simulink model "autopilot_vtolsim"  (R2019a)
settings: Solver=ode15s  StartTime=0.0  StopTime=10000  RelTol=1e-3  EnableMultiTasking=on
InitFcn:
  | clear all
  | path(pathdef)
  | addpath('.')
  | simulation_parameters
  | wind_parameters
undefined symbols (not defined in the file or in its folder): AP, autopilot, drawAircraft, Earth, forces_moments, plotvtolstatevariables, SIM, true_states, vtol, WGS84, WIND
libraries: simulink x3, aerolibfltsims x2, aerolibtransform2 x1
settings Model: Creator=beard  LastModifiedBy=nikhil
settings DataIOCC: LimitDataPoints=on  SaveFormat=Array  SignalLoggingSaveFormat=ModelDataLogs  ReturnWorkspaceOutputs=off
settings OptimizationCC: ExpressionDepthLimit=2147483647  InitFltsAndDblsToZero=on  LifeSpan=inf
settings DebuggingCC: UnderspecifiedInitializationDetection=Classic  MergeDetectMultiDrivingBlocksExec=none  SolverPrmCheckMsg=warning  FcnCallInpInsideContextMsg=warning  AllowSymbolicDim=off  StateNameClashWarn=warning  PregeneratedLibrarySubsystemCodeDiagnostic=none  SFUnexpectedBacktrackingDiag=warning  SFNoUnconditionalDefaultTransitionDiag=warning  SFExecutionAtInitializationDiag=none  ArithmeticOperatorsInVariantConditions=warning
settings HardwareCC: ProdBitPerPointer=32  ProdBitPerSizeT=32  ProdBitPerPtrDiffT=32  ProdLargestAtomicFloat=None  ProdIntDivRoundTo=Undefined  ProdEndianess=Unspecified  ProdWordSize=32  ProdHWDeviceType=32-bit Generic
settings ModelReferenceCC: PropagateSignalLabelsOutOfModel=off
settings SFSimCC: SimUseLocalCustomCode=off
settings RTWCC: RTWUseLocalCustomCode=off
settings CodeAppCC: StateflowObjectComments=on
settings GRTTargetCC: TargetLangStandard=C89/C90 (ANSI)  GeneratePreprocessorConditionals=Disable all  CombineOutputUpdateFcns=off  GRTInterface=on
settings ConfigComp: CovMetricSettings=dw  CovHtmlReporting=on  CovSaveCumulativeToWorkspaceVar=on  CovSaveSingleToWorkspaceVar=on  CovExternalEMLEnable=off  CovSFcnEnable=off

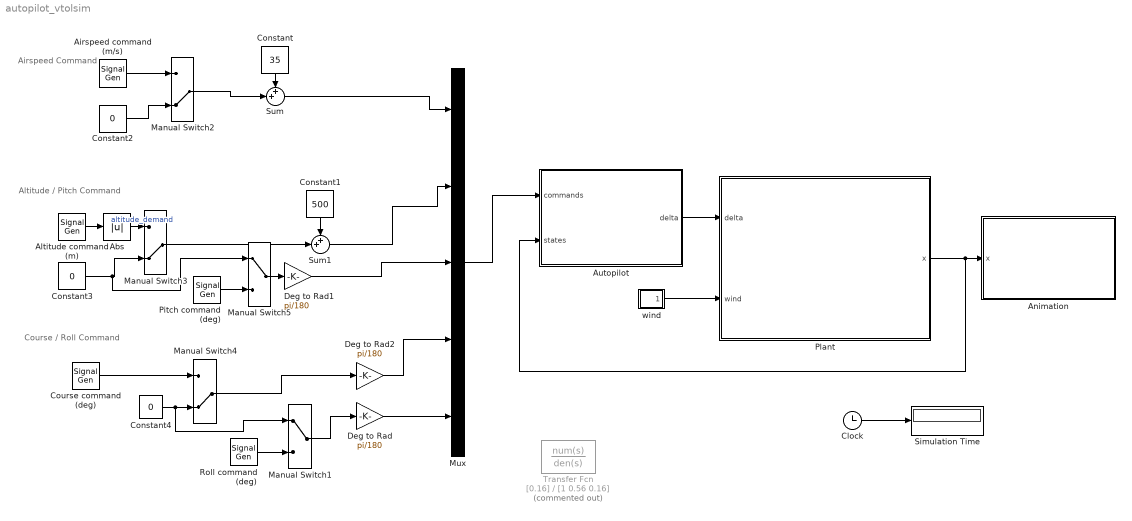
== system autopilot_vtolsim ==
  note: Airspeed Command
  note: Altitude / Pitch Command
  note: Course / Roll Command
  Abs : Abs
  Airspeed command (m/s) : SignalGenerator  WaveForm=square  Amplitude=5  Frequency=0.012
  Altitude command (m) : SignalGenerator  Amplitude=15  Frequency=.02
  Animation : Subsystem
      mask Display: image(imread('animation.jpg'))
  Autopilot : Subsystem
      mask Display: image(imread('stm32.jpg'))
  Clock : Clock
  Constant : Constant  Value=35
  Constant1 : Constant  Value=500
  Constant2 : Constant  Value=0
  Constant3 : Constant  Value=0
  Constant4 : Constant  Value=0
  Course command (deg) : SignalGenerator  Amplitude=45  Frequency=.012
  Deg to Rad : Gain  Gain=pi/180
  Deg to Rad1 : Gain  Gain=pi/180
  Deg to Rad2 : Gain  Gain=pi/180
  Manual Switch1 : ManualSwitch
  Manual Switch2 : ManualSwitch  CurrentSetting=0
  Manual Switch3 : ManualSwitch  CurrentSetting=0
  Manual Switch4 : ManualSwitch  CurrentSetting=0
  Manual Switch5 : ManualSwitch
  Mux : Mux  Inputs=5
  Pitch command (deg) : SignalGenerator  Amplitude=20  Frequency=0.1
  Plant : Subsystem
      mask Display: image(imread('vtol.jpeg'))
  Roll command (deg) : SignalGenerator  WaveForm=square  Amplitude=45  Frequency=.1
  Simulation Time : Display
  Sum : Sum  Inputs=++|
  Sum1 : Sum  Inputs=++|
  Transfer Fcn : TransferFcn  Commented=on  Numerator=[0.16]  Denominator=[1 0.56 0.16]
  wind : Subsystem
  wires:
  Clock/1 -> Simulation Time/1
  wind/1(Wind) -> Plant/2(wind)
  Plant/1(x) -> Autopilot/2(states), Animation/1(x)
  Autopilot/1(delta) -> Plant/1(delta)
  Deg to Rad/1 -> Mux/5
  Sum/1 -> Mux/1
  Constant/1 -> Sum/1
  Sum1/1 -> Mux/2
  Constant1/1 -> Sum1/1
  Deg to Rad1/1 -> Mux/3
  Airspeed command (m/s)/1 -> Manual Switch2/1
  Constant2/1 -> Manual Switch2/2
  Manual Switch3/1 -> Sum1/2
  Constant3/1 -> Manual Switch5/1, Manual Switch3/2
  Constant4/1 -> Manual Switch1/1, Manual Switch4/2
  Manual Switch4/1 -> Deg to Rad2/1
  Course command (deg)/1 -> Manual Switch4/1
  Manual Switch2/1 -> Sum/2
  Deg to Rad2/1 -> Mux/4
  Mux/1 -> Autopilot/1(commands)
  Roll command (deg)/1 -> Manual Switch1/2
  Manual Switch1/1 -> Deg to Rad/1
  Manual Switch5/1 -> Deg to Rad1/1
  Pitch command (deg)/1 -> Manual Switch5/2
  Altitude command (m)/1 -> Abs/1
  Abs/1 -> Manual Switch3/1  "altitude_demand"

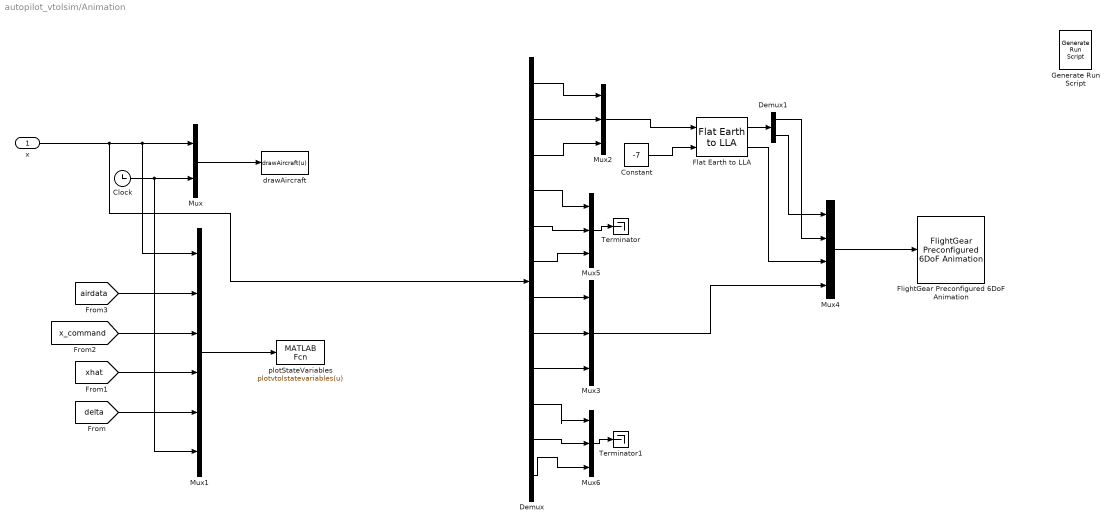
== system autopilot_vtolsim/Animation ==
  x : Inport
  Clock : Clock
  Constant : Constant  Value=-7
  Demux : Demux  Outputs=12
  Demux1 : Demux  Outputs=2
  Flat Earth to LLA : aerolibtransform2/Flat Earth to LLA  units=Metric (MKS)  ptype=Earth (WGS84)  F=1/298.257223563  R=6378137  LL0=[37.6188056,-122.3754167 ]  psi=0
  FlightGear Preconfigured 6DoF Animation : aerolibfltsims/FlightGear Preconfigured 6DoF Animation  xFlightGearVersion=v2018.2  DestinationIpAddress=127.0.0.1  DestinationPort=5502  SampleTime=1/30  packetVersion=24
      settings: SourceProductName=Aerospace Blockset
  Generate Run Script : aerolibfltsims/Generate Run Script  Architecture=Win64  dataFlow=Send  GeometryModelName=c172p  AirportId=KSFO  RunwayId=10L  InitialAltitude=0  InitialHeading=113  OffsetDistance=4.72  OffsetAzimuth=0  InstallScenery=on  DisableShaders=off  OriginAddress=127.0.0.1  DestinationPort=5502  OriginPort=5505  LocalAddress=127.0.0.1  OutputFileName=runfg.bat  FlightGearBaseDirectory=C:\Program Files\FlightGear 2019.1.1
  Mux : Mux  Inputs=2
  Mux1 : Mux  Inputs=6
  Mux{2..3,5..6} (4 alike) : Mux  Inputs=3
  Mux4 : Mux
  Terminator : Terminator
  Terminator1 : Terminator
  drawAircraft : MATLABFcn  MATLABFcn=drawAircraft(u)  OutputDimensions=0  SampleTime=SIM.ts_plotting
  plotStateVariables : MATLABFcn  MATLABFcn=plotvtolstatevariables(u)  OutputDimensions=0  SampleTime=SIM.ts_plotting
  wires:
  Mux/1 -> drawAircraft/1
  x/1 -> Demux/1, Mux/1, Mux1/1
  Clock/1 -> Mux/2, Mux1/6
  Mux1/1 -> plotStateVariables/1
  [xhat] -> Mux1/4
  [x_command] -> Mux1/3
  [delta] -> Mux1/5
  [airdata] -> Mux1/2
  Demux/1 -> Mux2/1
  Demux/2 -> Mux2/2
  Demux/3 -> Mux2/3
  Mux2/1 -> Flat Earth to LLA/1
  Constant/1 -> Flat Earth to LLA/2
  Demux/4 -> Mux5/1
  Demux/5 -> Mux5/2
  Demux/6 -> Mux5/3
  Demux/7 -> Mux3/1
  Demux/8 -> Mux3/2
  Demux/9 -> Mux3/3
  Demux/10 -> Mux6/1
  Demux/11 -> Mux6/2
  Demux/12 -> Mux6/3
  Flat Earth to LLA/1 -> Demux1/1
  Demux1/1 -> Mux4/2
  Demux1/2 -> Mux4/1
  Flat Earth to LLA/2 -> Mux4/3
  Mux3/1 -> Mux4/4
  Mux4/1 -> FlightGear Preconfigured 6DoF Animation/1
  Mux5/1 -> Terminator/1
  Mux6/1 -> Terminator1/1

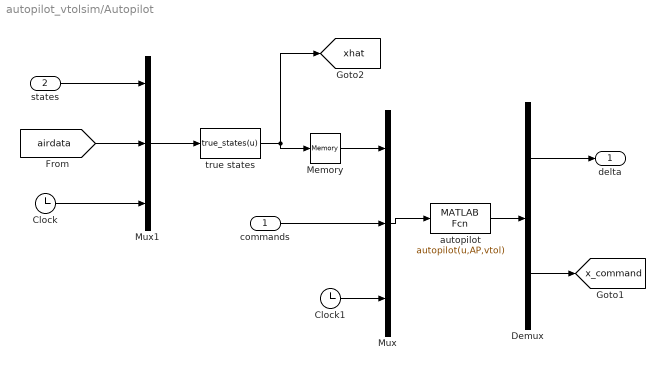
== system autopilot_vtolsim/Autopilot ==
  commands : Inport
  states : Inport  Port=2
  Clock : Clock
  Clock1 : Clock
  Demux : Demux  Outputs=[4;12]
  Memory : Memory  InheritSampleTime=on  LinearizeAsDelay=on
  Mux : Mux  Inputs=3
  Mux1 : Mux  Inputs=3
  autopilot : MATLABFcn  MATLABFcn=autopilot(u,AP,vtol)  OutputDimensions=4+12  SampleTime=SIM.ts_simulation
  true states : MATLABFcn  MATLABFcn=true_states(u)  OutputDimensions=19  SampleTime=SIM.ts_simulation
  delta : Outport
  tag scope: x_command=global, xhat=global
  wires:
  Mux/1 -> autopilot/1
  Clock/1 -> Mux1/3
  autopilot/1 -> Demux/1
  Demux/1 -> delta/1
  Demux/2 -> [x_command]
  commands/1 -> Mux/2
  Mux1/1 -> true states/1
  states/1 -> Mux1/1
  true states/1 -> [xhat], Memory/1
  [airdata] -> Mux1/2
  Memory/1 -> Mux/1
  Clock1/1 -> Mux/3

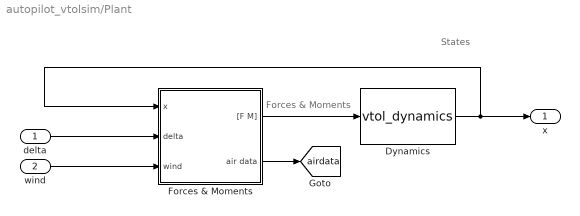
== system autopilot_vtolsim/Plant ==
  note: Forces & Moments
  note: States
  delta : Inport
  wind : Inport  Port=2
  Dynamics : S-Function  InitFcn=|  FunctionName=vtol_dynamics  Parameters=vtol  SFunctionDeploymentMode=off  EnableBusSupport=off
      | addpath('.')
      | simulation_parameters
      | vtol_parameters
  Forces & Moments : Subsystem
  x : Outport
  tag scope: airdata=global
  wires:
  Dynamics/1 -> Forces & Moments/1(x), x/1
  Forces & Moments/1("[F M]") -> Dynamics/1
  Forces & Moments/2(air data) -> [airdata]
  delta/1 -> Forces & Moments/2(delta)
  wind/1 -> Forces & Moments/3(wind)

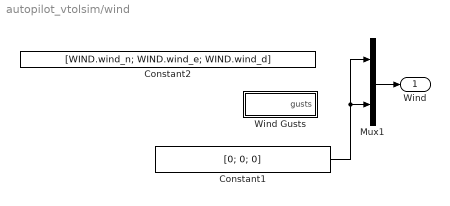
== system autopilot_vtolsim/wind ==
  Constant1 : Constant  Value=[0; 0; 0]
  Constant2 : Constant  Value=[WIND.wind_n; WIND.wind_e; WIND.wind_d]
  Mux1 : Mux  Inputs=2
  Wind Gusts : Subsystem
  Wind : Outport
  wires:
  Mux1/1 -> Wind/1
  Constant1/1 -> Mux1/2, Mux1/1

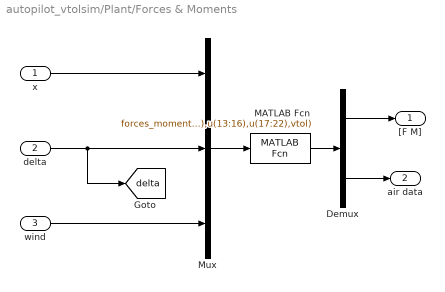
== system autopilot_vtolsim/Plant/Forces & Moments ==
  x : Inport
  delta : Inport  Port=2
  wind : Inport  Port=3
  Demux : Demux  Outputs=[6;6]
  MATLAB Fcn : MATLABFcn  MATLABFcn=forces_moments(u(1:12),u(13:16),u(17:22),vtol)  OutputDimensions=12
  Mux : Mux  Inputs=3
  "[F M]" : Outport
  air data : Outport  Port=2
  tag scope: delta=global
  wires:
  Demux/2 -> air data/1
  Mux/1 -> MATLAB Fcn/1
  Demux/1 -> "[F M]"/1
  MATLAB Fcn/1 -> Demux/1
  wind/1 -> Mux/3
  delta/1 -> Mux/2, [delta]
  x/1 -> Mux/1

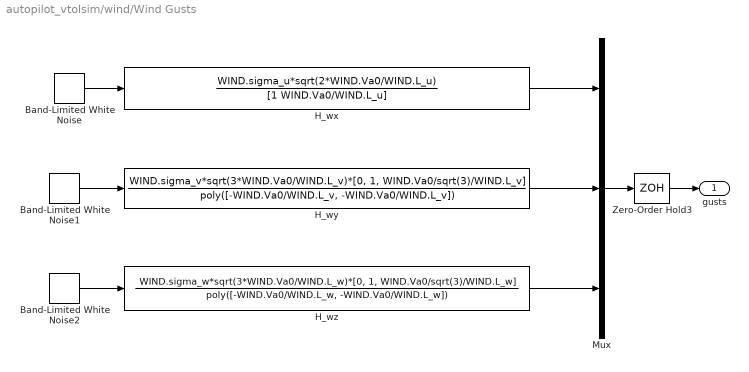
== system autopilot_vtolsim/wind/Wind Gusts ==
  Band-Limited White Noise : simulink/Sources/Band-Limited White Noise  Cov=[1]  Ts=SIM.ts_simulation  seed=[23341]
  Band-Limited White Noise1 : simulink/Sources/Band-Limited White Noise  Cov=[1]  Ts=SIM.ts_simulation  seed=[23341]
  Band-Limited White Noise2 : simulink/Sources/Band-Limited White Noise  Cov=[1]  Ts=SIM.ts_simulation  seed=[23341]
  H_wx : TransferFcn  Numerator=WIND.sigma_u*sqrt(2*WIND.Va0/WIND.L_u)  Denominator=[1 WIND.Va0/WIND.L_u]
  H_wy : TransferFcn  Numerator=WIND.sigma_v*sqrt(3*WIND.Va0/WIND.L_v)*[0, 1, WIND.Va0/sqrt(3)/WIND.L_v]  Denominator=poly([-WIND.Va0/WIND.L_v, -WIND.Va0/WIND.L_v])
  H_wz : TransferFcn  Numerator=WIND.sigma_w*sqrt(3*WIND.Va0/WIND.L_w)*[0, 1, WIND.Va0/sqrt(3)/WIND.L_w]  Denominator=poly([-WIND.Va0/WIND.L_w, -WIND.Va0/WIND.L_w])
  Mux : Mux  Inputs=3
  Zero-Order Hold3 : ZeroOrderHold  SampleTime=SIM.ts_simulation
  gusts : Outport
  wires:
  H_wx/1 -> Mux/1
  Band-Limited White Noise/1 -> H_wx/1
  H_wy/1 -> Mux/2
  Band-Limited White Noise1/1 -> H_wy/1
  H_wz/1 -> Mux/3
  Band-Limited White Noise2/1 -> H_wz/1
  Mux/1 -> Zero-Order Hold3/1
  Zero-Order Hold3/1 -> gusts/1
